simulink model "SinglephaseDualConverter"  (Simulink 7.3)
settings: Solver=ode45  StartTime=0.0  StopTime=5  RelTol=1e-3
libraries: powerlib x15
settings Model: Creator=srija  LastModifiedBy=srija

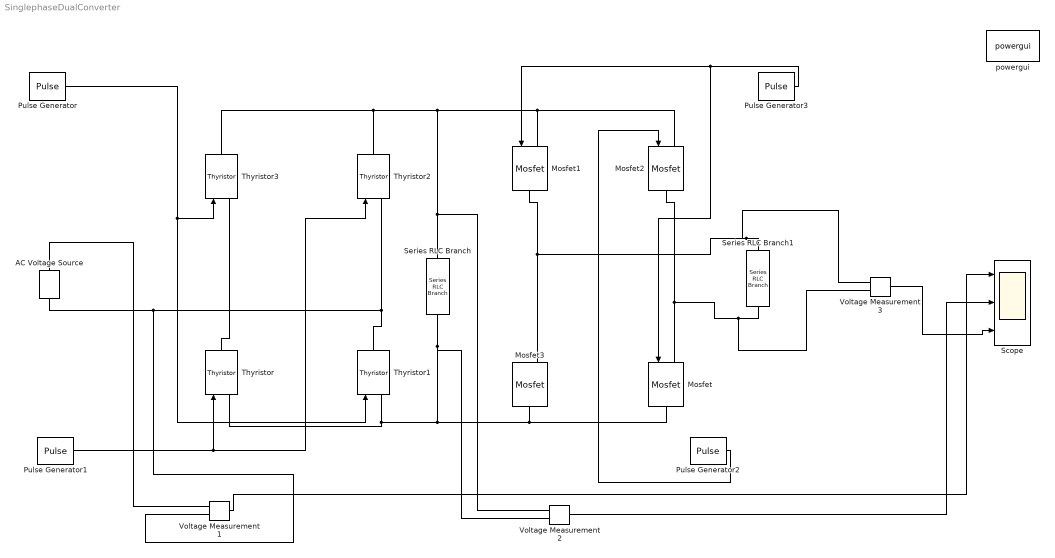
== system SinglephaseDualConverter ==
  AC Voltage Source : powerlib/Electrical Sources/AC Voltage Source  DialogController=POWERSYS.PowerSysDialog  SystemSampleTime=-1  Amplitude=300  Phase=0  Frequency=50  SampleTime=0  Measurements=None
  Mosfet{,1..3} (4 alike) : powerlib/Power Electronics/Mosfet  DialogController=POWERSYS.PowerSysDialog  SystemSampleTime=-1  Ron=0.1  Lon=0  Rd=0.01  Vfd=0  IC=0  Rs=1e5  Cs=inf  Measurements=off
  Pulse Generator{,1..3} (4 alike) : DiscretePulseGenerator  PulseType=Time based  Amplitude=5  Period=0.02  PulseWidth=50  PhaseDelay=0.016  SampleTime=1
  Scope : Scope  NumInputPorts=3
      settings: TimeRange=5  YMin=-5~-5~-5  YMax=5~5~5
  Series RLC Branch : powerlib/Elements/Series RLC Branch  DialogController=POWERSYS.PowerSysDialog  PhysicalDomain=powersysdomain  SubClassName=unknown  LeftPortType=p1  RightPortType=p1  LConnTagsString=__new0  RConnTagsString=__new0  BranchType=R  Resistance=300  Inductance=1e-3  SetiL0=off  InitialCurrent=0  Capacitance=1e-6  Setx0=off  InitialVoltage=0  Measurements=Branch voltage
  Series RLC Branch1 : powerlib/Elements/Series RLC Branch  DialogController=POWERSYS.PowerSysDialog  PhysicalDomain=powersysdomain  SubClassName=unknown  LeftPortType=p1  RightPortType=p1  LConnTagsString=__new0  RConnTagsString=__new0  BranchType=R  Resistance=700  Inductance=1e-3  SetiL0=off  InitialCurrent=0  Capacitance=1e-6  Setx0=off  InitialVoltage=0  Measurements=Branch voltage
  Thyristor{,1..3} (4 alike) : powerlib/Power Electronics/Thyristor  DialogController=POWERSYS.PowerSysDialog  SystemSampleTime=-1  Ron=0.001  Lon=0  Vf=0.8  IC=0  Rs=500  Cs=250e-9  Measurements=off
  Voltage Measurement1 : powerlib/Measurements/Voltage Measurement  DialogController=POWERSYS.PowerSysDialog  SystemSampleTime=-1  PhasorSimulation=off  OutputType=Complex  PSBequivalent=0
  Voltage Measurement2 : powerlib/Measurements/Voltage Measurement  DialogController=POWERSYS.PowerSysDialog  SystemSampleTime=-1  PhasorSimulation=off  OutputType=Complex  PSBequivalent=0
  Voltage Measurement3 : powerlib/Measurements/Voltage Measurement  DialogController=POWERSYS.PowerSysDialog  SystemSampleTime=-1  PhasorSimulation=off  OutputType=Complex  PSBequivalent=0
  powergui : powerlib/powergui  Priority=1  SystemSampleTime=-1  SimulationMode=Continuous  SampleTime=50e-6  frequency=60  SPID=off  DisableSnubberDevices=off  DisableRonSwitches=off  DisableVfSwitches=off  SwTol=0  Interpol=off  frequencyindice=50  echomessages=off  HookPort=off  DisplayEquations=off  FunctionMessages=off  EnableUseOfTLC=off  x0status=blocks  RestoreLinks=warning  Frange=[0:2:500]  Ylog=off  Xlog=on  ShowGrid=off  save=off  variable=ZData  ZoomFFT=on  StartTime=0.0  cycles=1  DisplayStyle=1  fundamental=60  FreqAxis=off  MaxFrequency=1000  frequencyindicesteady=1  RmsSteady=1  display=off  Ts=0  methode=off
  wires:
  Pulse Generator/1 -> Thyristor1/1, Thyristor3/1
  Pulse Generator1/1 -> Thyristor2/1, Thyristor/1
  Voltage Measurement1/1 -> Scope/1
  Pulse Generator3/1 -> Mosfet1/1, Mosfet/1
  Pulse Generator2/1 -> Mosfet2/1
  Voltage Measurement2/1 -> Scope/2
  Voltage Measurement3/1 -> Scope/3
  connections:
  AC Voltage Source/RConn1 -- Voltage Measurement1/LConn1
  Thyristor3/LConn1 -- Thyristor/RConn1
  Mosfet3/RConn1 -- Series RLC Branch/RConn1 -- Voltage Measurement2/LConn2 -- Thyristor1/LConn1 -- Thyristor/LConn1 -- Mosfet/RConn1
  Thyristor1/RConn1 -- Thyristor2/LConn1 -- AC Voltage Source/LConn1 -- Voltage Measurement1/LConn2
  Thyristor3/RConn1 -- Thyristor2/RConn1 -- Mosfet2/LConn1 -- Mosfet1/LConn1 -- Series RLC Branch/LConn1 -- Voltage Measurement2/LConn1
  Mosfet1/RConn1 -- Mosfet3/LConn1 -- Series RLC Branch1/LConn1 -- Voltage Measurement3/LConn1
  Series RLC Branch1/RConn1 -- Mosfet2/RConn1 -- Mosfet/LConn1 -- Voltage Measurement3/LConn2
